simulink model "DinamicaCovid"  (R2021b)
settings: Solver=VariableStepAuto  StartTime=0.0  StopTime=100  MaxStep=1  MinStep=1  RelTol=1e-3
values from neighbouring files (symbols this model uses):
  I0 = 1    [ErroQuadraticoVini.m]
  r = X(1)    [ErroQuadraticoVini.m]
  R0 = 0    [ErroQuadraticoVini.m]
  S0 = 499    [ErroQuadraticoVini.m]
undefined symbols (not defined in the file or in its folder): Beta
settings Model: Creator=20.00134-7  LastModifiedBy=20.00134-7

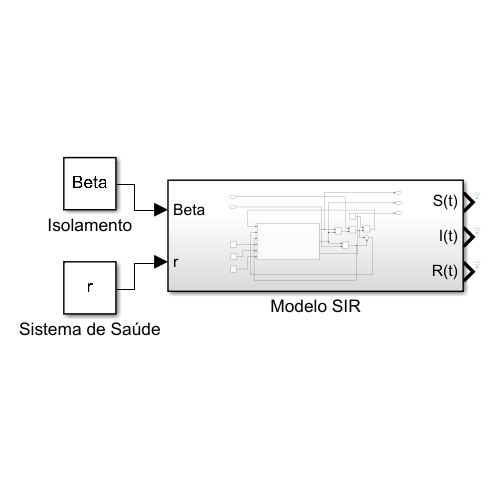
[thumbnail: Simulink's stored preview of the top-level diagram]
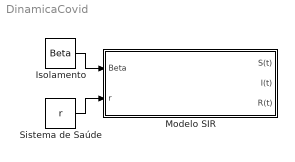
== system DinamicaCovid ==
  Isolamento : Constant  Value=Beta
  Modelo SIR : Subsystem
  Sistema de Saúde : Constant  Value=r
  wires:
  Isolamento/1 -> Modelo SIR/1(Beta)
  Sistema de Saúde/1 -> Modelo SIR/2(r)

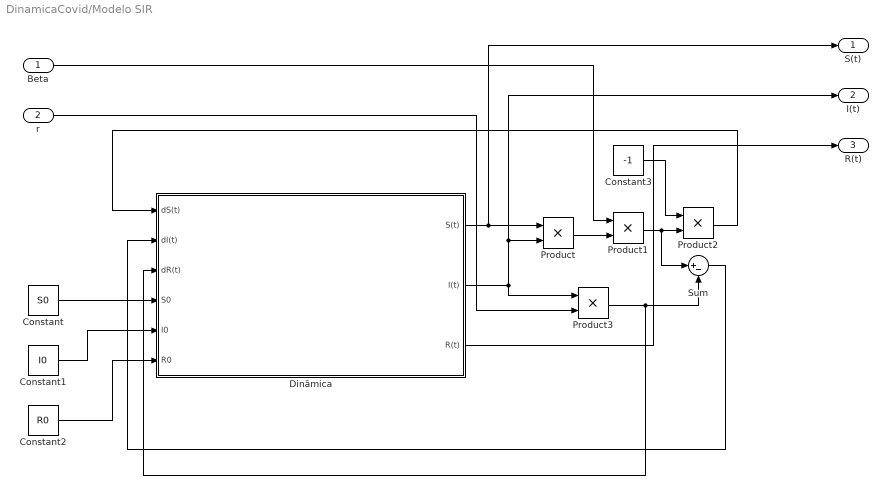
== system DinamicaCovid/Modelo SIR ==
  Beta : Inport
  r : Inport  Port=2
  Constant : Constant  Value=S0
  Constant1 : Constant  Value=I0
  Constant2 : Constant  Value=R0
  Constant3 : Constant  Value=-1
  Dinâmica : Subsystem
  Product{,1..3} (4 alike) : Product
  Sum : Sum  Inputs=|+-
  S(t) : Outport
  I(t) : Outport  Port=2
  R(t) : Outport  Port=3
  wires:
  Dinâmica/2(I(t)) -> I(t)/1, Product/2, Product3/1
  Beta/1 -> Product1/1
  Constant1/1 -> Dinâmica/5(I0)
  Product3/1 -> Dinâmica/3(dR(t)), Sum/2
  Dinâmica/1(S(t)) -> S(t)/1, Product/1
  Product2/1 -> Dinâmica/1(dS(t))
  Constant2/1 -> Dinâmica/6(R0)
  Product1/1 -> Product2/2, Sum/1
  r/1 -> Product3/2
  Sum/1 -> Dinâmica/2(dI(t))
  Constant/1 -> Dinâmica/4(S0)
  Dinâmica/3(R(t)) -> R(t)/1
  Product/1 -> Product1/2
  Constant3/1 -> Product2/1

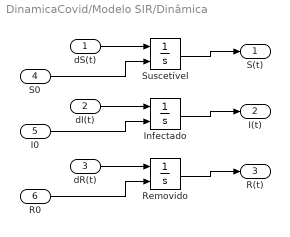
== system DinamicaCovid/Modelo SIR/Dinâmica ==
  dS(t) : Inport
  dI(t) : Inport  Port=2
  dR(t) : Inport  Port=3
  S0 : Inport  Port=4
  I0 : Inport  Port=5
  R0 : Inport  Port=6
  Infectado : Integrator  InitialConditionSource=external
  Removido : Integrator  InitialConditionSource=external
  Suscetível : Integrator  InitialConditionSource=external
  S(t) : Outport
  I(t) : Outport  Port=2
  R(t) : Outport  Port=3
  wires:
  Infectado/1 -> I(t)/1
  dS(t)/1 -> Suscetível/1
  R0/1 -> Removido/2
  dR(t)/1 -> Removido/1
  Removido/1 -> R(t)/1
  dI(t)/1 -> Infectado/1
  S0/1 -> Suscetível/2
  Suscetível/1 -> S(t)/1
  I0/1 -> Infectado/2
